simulink library "ddm"  (R2021b)
settings: Solver=VariableStepAuto  StartTime=0.0  StopTime=10.0  RelTol=1e-3
undefined symbols (not defined in the file): ADDM_FrTMTqDev_X_Nm, ADDM_RrTMTqDev_X_Nm, ENUM_ADASACCSTA_ERROR, ENUM_ADASACCSTA_OFF, ENUM_ADASACCSTA_STANDBY, ENUM_ALLOWMOV_ALLOWREADY, ENUM_APS, ENUM_BRKSTA_ERROR, ENUM_BRKSTA_OFF, ENUM_BRKSTA_ON, ENUM_BRKSW_INVALID, ENUM_BRKSW_OFF, ENUM_BRKSW_ON, ENUM_CHGPREACTERRSTA_OBCPRE, ENUM_DCDCFAULTSTA_ANYFAULTLV1, ENUM_DCDCFAULTSTA_ANYFAULTLV2, ENUM_DRIVETRAIN_AWD, ENUM_DRIVETRAIN_FWD, ENUM_DRIVETRAIN_RWD, ENUM_EDUDRTSTA_NORMAL, ENUM_EPBERROR_FAILED, ENUM_EPBSTA_APPLIED, ENUM_EPBSTA_RELEASED, ENUM_ESCAPSSta_APSUNAVAILABLE, ENUM_GEARACTUALPOSN_INVALID, ENUM_GEARACTUALPOSN_P, ENUM_HVBATTREADYPRE_READY, ENUM_HWRESETSTA_HWRESETING, ENUM_MCUWARN_LV0, ENUM_MCUWARN_LV1, ENUM_MCUWARN_LV2, ENUM_MCUWARN_LV3, ENUM_MCUWARN_NOERROR, ENUM_OBCFAULTSTA_ANYFAULT, ENUM_PAS_R2F2, ENUM_PDFAULT_BATTPDFAIL, ENUM_PDFAULT_DCDCDISABLE, ENUM_PDFAULT_MCUDISABLE, ENUM_PDFAULT_MCUDISCHRG, ENUM_POWERSTA_OFF, ENUM_POWERSTA_ON, ENUM_POWERSTA_READY, ENUM_POWERSTA_STANDBY, ENUM_PRESSINDI_LOW, ENUM_PUFAULT_BATTUPFAIL, ENUM_PUFAULT_DCDCENABLEFAIL, ENUM_PUFAULT_PRECHRGCHKFAIL, ENUM_PUFAULT_SAFETYCHKFAIL, ENUM_PWRSTASW_OFF, ENUM_PWRSTASW_OFFA, ENUM_PWRSTASW_OFFCHVCHRG, ENUM_PWRSTASW_OFFCLVCHRG, ENUM_PWRSTASW_ON, ENUM_PWRSTASW_ONHVCHRG, ENUM_PWRSTASW_READY, ENUM_PWRSTASW_STANDBY, ENUM_RAPSErrWarnSta_NORMAL, ENUM_RAPSErrWarnSta_RAPSERRLV1, ENUM_SHIFTCOMMAND_P, ENUM_SHIFTERERRSTA_PBUTTONFAILURE ... (+471)
libraries: hcu_lib x540, simulink x3
(part 7 of 26)

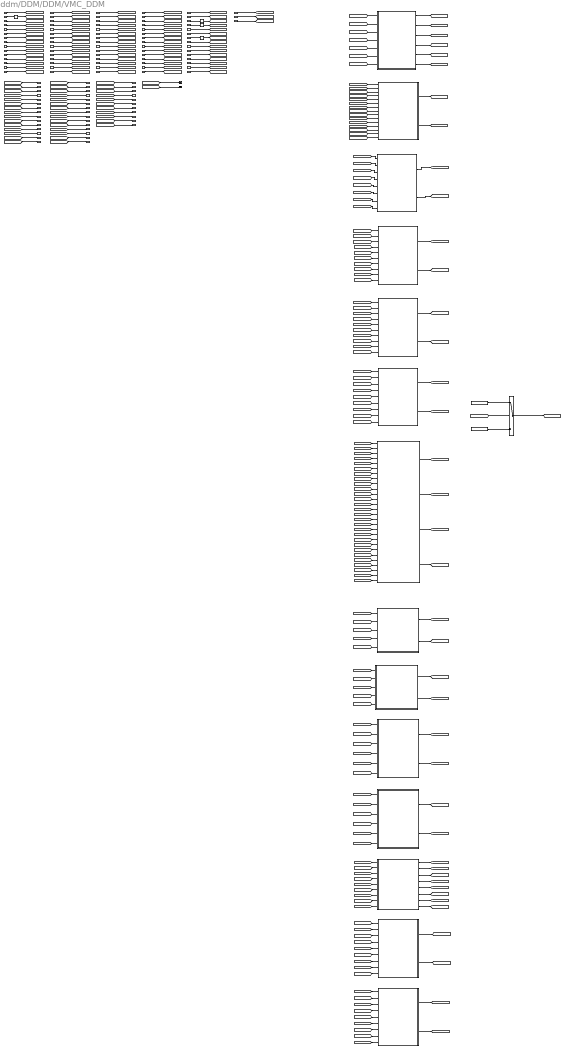
== system ddm/DDM/DDM/VMC_DDM ==
  note: No_CAN3_BUS_OFF
  note: ACC Accel
  note: CCU
  note: MCU_Rr
  note: MCU_Fr
  note: FCMACC
  note: BMS
  note: FCM1
  note: Shifter
  note: ESC
  note: Zone_dr VCU
  note: Zone_fr VCU
  note: Zone_dr
  note: Zone_fr
  note: EPS1
  task_time_s : Inport
  VDDM_FCM1NoCom_flg : Inport  Port=2
  VDDM_FCM1RCErr_flg : Inport  Port=3
  VDDM_FCM1CSErr_flg : Inport  Port=4
  VPMM_PowerSta_enum : Inport  Port=5
  VINP_ADASACCSta_enum : Inport  Port=6
  DTC_clear_request : Inport  Port=7
  VDDM_C3BMS6LCCFS_flg : Inport  Port=8
  VDDM_C3BMS6RCCFS_flg : Inport  Port=9
  VDDM_C3BMS6CSCFS_flg : Inport  Port=10
  VINP_BMSWarn8_flg : Inport  Port=11
  VINP_BMSWarn7_flg : Inport  Port=12
  VINP_BMSWarn6_flg : Inport  Port=13
  VINP_BMSWarn5_flg : Inport  Port=14
  VINP_BMSWarn4_flg : Inport  Port=15
  VINP_BMSWarn3_flg : Inport  Port=16
  VINP_VehSpeed_kph : Inport  Port=17
  VDDM_MCUF1NoComCFS_flg : Inport  Port=18
  VDDM_MCUF1RCErrCFS_flg : Inport  Port=19
  VDDM_MCUF1CSErrCFS_flg : Inport  Port=20
  VDDM_MCUWarnF_enum : Inport  Port=21
  VDDM_MCUWarnR_enum : Inport  Port=22
  VDDM_MCUR1NoComCFS_flg : Inport  Port=23
  VDDM_MCUR1RCErrCFS_flg : Inport  Port=24
  VDDM_MCUR1CSErrCFS_flg : Inport  Port=25
  VDDM_C3CCU2LCCFS_flg : Inport  Port=26
  VDDM_C3CCU2RCCFS_flg : Inport  Port=27
  VDDM_C3CCU2CSCFS_flg : Inport  Port=28
  VINP_DCDCFaultSta_enum : Inport  Port=29
  VVMC_ADASActive_flg : Inport  Port=30
  VINP_ACCRequireAccel_mps2 : Inport  Port=31
  VDDM_ESC1Err_flg : Inport  Port=32
  VDDM_ESC5Err_flg : Inport  Port=33
  VINP_ZoneSpdCtrlMode_enum : Inport  Port=34
  No_CAN1_BUS_OFF : Inport  Port=35
  No_CAN3_BUS_OFF : Inport  Port=36
  No_CAN4_BUS_OFF : Inport  Port=37
  No_CAN6_BUS_OFF : Inport  Port=38
  VTQD_ExternalTqAllow_flg : Inport  Port=39
  VTQD_ExtDoorAllow_flg : Inport  Port=40
  VINP_BMSWarn2_flg : Inport  Port=41
  VINP_BMSWarn1_flg : Inport  Port=42
  VDDM_Shifter1NoComCFS_flg : Inport  Port=43
  VDDM_Shifter1RCErrCFS_flg : Inport  Port=44
  VDDM_Shifter1CSErrCFS_flg : Inport  Port=45
  VINP_ShifterFailsta_enum : Inport  Port=46
  VTQD_GearActualPosn_enum : Inport  Port=47
  VINP_ABSFailed_flg : Inport  Port=48
  VINP_TCSFailed_flg : Inport  Port=49
  VINP_ESCFailed_flg : Inport  Port=50
  VINP_HSAFailed_flg : Inport  Port=51
  VINP_AVHFailed_flg : Inport  Port=52
  VINP_MCPressureV_flg : Inport  Port=53
  VINP_BrkSwV_flg : Inport  Port=54
  VINP_BrkPedalPosSta_flg : Inport  Port=55
  VINP_LongAccelV_flg : Inport  Port=56
  VINP_LatAccelV_flg : Inport  Port=57
  VINP_YawRateV_flg : Inport  Port=58
  VINP_LRRawWhlSpeedV_flg : Inport  Port=59
  VINP_RRRawWhlSpeedV_flg : Inport  Port=60
  VINP_LFRawWhlSpeedV_flg : Inport  Port=61
  VINP_RFRawWhlSpeedV_flg : Inport  Port=62
  VINP_CANMsgValidZoneDrVCU_flg : Inport  Port=63
  VINP_CANMsgValidZoneFrVCU_flg : Inport  Port=64
  VINP_ZoneDrMalfunLevel_enum : Inport  Port=65
  ZoneFrMalfunLevel_enum : Inport  Port=66
  VINP_CANMsgValidEPS1_flg : Inport  Port=67
  VDDM_EPSRCErr_flg : Inport  Port=68
  VDDM_EPSCSErr_flg : Inport  Port=69
  VINP_SASV_flg : Inport  Port=70
  VPMM_DrivetrainSelect_enum : Inport  Port=71
  VDDM_ClearZevDTCcmd_flg : Inport  Port=72
  VINP_FrntAxlTrqReqDrv_Nm : Inport  Port=73
  VINP_RearAxlTrqReqDrv_Nm : Inport  Port=74
  VINP_GRADE_Deg : Inport  Port=75
  VINP_FrntAxlTrqReqBrk_Nm : Inport  Port=76
  VINP_RearAxlTrqReqBrk_Nm : Inport  Port=77
  VINP_ESCAPSSta_enum : Inport  Port=78
  ACC Acceleration Command Error : Subsystem
  "BMS Signal Error " : Subsystem
  CCU Signal Error : Subsystem
  Constant4 : Constant  Value=TRUE
  Constant5 : Constant  Value=FALSE
  ESC Signal Error : Subsystem
  Enabled Subsystem : Subsystem  TreatAsAtomicUnit=on
  FCM1 : Subsystem
  FCMACC Signal Error : Subsystem
  Logical Operator : Logic  Operator=NOT  AllPortsSameDT=off  OutDataTypeStr=boolean
  Logical Operator1 : Logic  Operator=NOT  AllPortsSameDT=off  OutDataTypeStr=boolean
  MCU_Fr Signal Error : Subsystem
  MCU_Rr Signal Error : Subsystem
  NOT1 : Logic  Operator=NOT  AllPortsSameDT=off  OutDataTypeStr=boolean
  NOT21 : Logic  Operator=NOT  AllPortsSameDT=off  OutDataTypeStr=boolean
  Shifter Signal Error : Subsystem
  Switch2 : Switch  Criteria=u2 ~= 0
  Terminator1 : Terminator
  Terminator2 : Terminator
  Zone_Dr_VCU : Subsystem
  Zone_Fr_VCU : Subsystem
  Zone_dr Error : Subsystem
  Zone_fr Error : Subsystem
  VDDM_FCM1NoComDTC_raw32 : Outport
  VDDM_FCM1RCErrDTC_raw32 : Outport  Port=2
  VDDM_FCM1CSErrDTC_raw32 : Outport  Port=3
  VDDM_BMSSigErrDetDTC_raw32 : Outport  Port=4
  VDDM_FCMACCSigErrDetDTC_raw32 : Outport  Port=5
  VDDM_CCUSigErrDetDTC_raw32 : Outport  Port=6
  VDDM_ACCAccelCmdErrDetDTC_raw32 : Outport  Port=7
  VDDM_ESCSigErrDetDTC_raw32 : Outport  Port=8
  VDDM_ShifterSigErrDetDTC_raw32 : Outport  Port=9
  VDDM_DrVCUNoComDTC_raw32 : Outport  Port=10
  VDDM_FrVCUNoComDTC_raw32 : Outport  Port=11
  VDDM_ZoneDrSigErrDetDTC_raw32 : Outport  Port=12
  VDDM_ZoneFrSigErrDetDTC_raw32 : Outport  Port=13
  VDDM_EPS1NoComDTC_raw32 : Outport  Port=14
  VDDM_EPS1RCErrDTC_raw32 : Outport  Port=15
  VDDM_EPS1CSErrDTC_raw32 : Outport  Port=16
  VDDM_EPSSigErrDTC_raw32 : Outport  Port=17
  VDDM_FrMCUSigErrDetDTC_raw32 : Outport  Port=18
  VDDM_RrMCUSigErrDetDTC_raw32 : Outport  Port=19
  VDDM_FCM1NoComCFS_flg : Outport  Port=20
  VDDM_FCM1RCErrCFS_flg : Outport  Port=21
  VDDM_FCM1CSErrCFS_flg : Outport  Port=22
  VDDM_BMSSigErrCFS_flg : Outport  Port=23
  VDDM_FCMACCSigErrCFS_flg : Outport  Port=24
  VDDM_CCUSigErrCFS_flg : Outport  Port=25
  VDDM_ACCAccelCmdErrCFS_flg : Outport  Port=26
  VDDM_ESCSigErrCFS_flg : Outport  Port=27
  VDDM_ShifterSigErrCFS_flg : Outport  Port=28
  VDDM_DrVCUNoComCFS_flg : Outport  Port=29
  VDDM_FrVCUNoComCFS_flg : Outport  Port=30
  VDDM_ZoneDrSigErrCFS_flg : Outport  Port=31
  VDDM_ZoneFrSigErrCFS_flg : Outport  Port=32
  VDDM_EPS1NoComCFS_flg : Outport  Port=33
  VDDM_EPS1RCErrCFS_flg : Outport  Port=34
  VDDM_EPS1CSErrCFS_flg : Outport  Port=35
  VDDM_EPSSigErrCFS_flg : Outport  Port=36
  VDDM_FrMCUSigErrCFS_flg : Outport  Port=37
  VDDM_RrMCUSigErrCFS_flg : Outport  Port=38
  VDDM_ESC1SigErr_flg : Outport  Port=39
  VDDM_ESC5SigErr_flg : Outport  Port=40
  VDDM_EDriveSysErrVCUErrVMC_flg : Outport  Port=41
  wires:
  CCU Signal Error/2(VDDM_CCUSigErrDetDTC_raw32) -> [VDDM_CCUSigErrDetDTC_raw32]
  MCU_Rr Signal Error/2(VDDM_RrMCUSigErrDetDTC_raw32) -> [VDDM_RrMCUSigErrDetDTC_raw32]
  "BMS Signal Error "/2(VDDM_BMSSigErrDetDTC_raw32) -> [VDDM_BMSSigErrDetDTC_raw32]
  No_CAN1_BUS_OFF/1 -> [No_CAN1_BUS_OFF]
  No_CAN3_BUS_OFF/1 -> [No_CAN3_BUS_OFF]
  No_CAN4_BUS_OFF/1 -> [No_CAN4_BUS_OFF]
  VINP_ZoneSpdCtrlMode_enum/1 -> [VINP_ZoneSpdCtrlMode_enum]
  VDDM_ESC5Err_flg/1 -> [VDDM_ESC5Err_flg]
  VDDM_ESC1Err_flg/1 -> [VDDM_ESC1Err_flg]
  VINP_ACCRequireAccel_mps2/1 -> [VINP_ACCRequireAccel_mps2]
  VVMC_ADASActive_flg/1 -> [VVMC_ADASActive_flg]
  [VINP_ADASACCSta_enum] -> ACC Acceleration Command Error/9(VINP_ADASACCSta_enum)
  [VVMC_ADASActive_flg] -> ACC Acceleration Command Error/5(VVMC_ADASActive_flg)
  ACC Acceleration Command Error/1(VDDM_ACCAccelCmdErrCFS_flg) -> [VDDM_ACCAccelCmdErrCFS_flg]
  [No_CAN6_BUS_OFF] -> ACC Acceleration Command Error/6(No_CAN6_BUS_OFF)
  [VPMM_PowerSta_enum] -> ACC Acceleration Command Error/7(VPMM_PowerSta_enum)
  [DTC_clear_request] -> ACC Acceleration Command Error/10(DTC_clear_request)
  [VDDM_FCM1NoComCFS_flg] -> ACC Acceleration Command Error/2(VDDM_FCM1NoComCFS_flg)
  [VINP_ACCRequireAccel_mps2] -> ACC Acceleration Command Error/8(VINP_ACCRequireAccel_mps2)
  [VDDM_FCM1RCErrCFS_flg] -> ACC Acceleration Command Error/3(VDDM_FCM1RCErrCFS_flg)
  [VDDM_FCM1CSErrCFS_flg] -> ACC Acceleration Command Error/4(VDDM_FCM1CSErrCFS_flg)
  [task_time_s] -> ACC Acceleration Command Error/1(task_time_s)
  VINP_DCDCFaultSta_enum/1 -> [VINP_DCDCFaultSta_enum]
  VDDM_C3CCU2CSCFS_flg/1 -> [VDDM_C3CCU2CSCFS_flg]
  VDDM_C3CCU2RCCFS_flg/1 -> [VDDM_C3CCU2RCCFS_flg]
  VDDM_C3CCU2LCCFS_flg/1 -> [VDDM_C3CCU2LCCFS_flg]
  CCU Signal Error/1(VDDM_CCUSigErrCFS_flg) -> [VDDM_CCUSigErrCFS_flg]
  [VDDM_C3CCU2LCCFS_flg] -> CCU Signal Error/2(VDDM_C3CCU2LCCFS_flg)
  [task_time_s] -> CCU Signal Error/1(task_time_s)
  [VINP_DCDCFaultSta_enum] -> CCU Signal Error/7(VINP_DCDCFaultSta_enum)
  [VDDM_C3CCU2RCCFS_flg] -> CCU Signal Error/3(VDDM_C3CCU2RCCFS_flg)
  [VDDM_C3CCU2CSCFS_flg] -> CCU Signal Error/4(VDDM_C3CCU2CSCFS_flg)
  [VDDM_ClearZevDTCcmd_flg] -> CCU Signal Error/8(DTC_clear_request)
  [VPMM_PowerSta_enum] -> CCU Signal Error/6(VPMM_PowerSta_enum)
  [No_CAN3_BUS_OFF] -> CCU Signal Error/5(No_CAN3_BUS_OFF)
  VDDM_MCUR1CSErrCFS_flg/1 -> [VDDM_MCUR1CSErrCFS_flg]
  VDDM_MCUR1RCErrCFS_flg/1 -> [VDDM_MCUR1RCErrCFS_flg]
  VDDM_MCUR1NoComCFS_flg/1 -> [VDDM_MCUR1NoComCFS_flg]
  VDDM_MCUWarnR_enum/1 -> [VDDM_MCUWarnR_enum]
  [task_time_s] -> MCU_Rr Signal Error/1(task_time_s)
  [VDDM_MCUR1RCErrCFS_flg] -> MCU_Rr Signal Error/3(VDDM_MCUR1RCErrCFS_flg)
  [VDDM_MCUR1NoComCFS_flg] -> MCU_Rr Signal Error/2(VDDM_MCUR1NoComCFS_flg)
  MCU_Rr Signal Error/1(VDDM_RrMCUSigErrCFS_flg) -> [VDDM_RrMCUSigErrCFS_flg]
  [VPMM_PowerSta_enum] -> MCU_Rr Signal Error/6(VPMM_PowerSta_enum)
  [VDDM_MCUWarnR_enum] -> MCU_Rr Signal Error/7(VDDM_MCUWarnR_enum)
  [VDDM_MCUR1CSErrCFS_flg] -> MCU_Rr Signal Error/4(VDDM_MCUR1CSErrCFS_flg)
  [VDDM_ClearZevDTCcmd_flg] -> MCU_Rr Signal Error/8(DTC_clear_request)
  [No_CAN3_BUS_OFF] -> MCU_Rr Signal Error/5(No_CAN3_BUS_OFF)
  VDDM_MCUWarnF_enum/1 -> [VDDM_MCUWarnF_enum]
  VDDM_MCUF1CSErrCFS_flg/1 -> [VDDM_MCUF1CSErrCFS_flg]
  VDDM_MCUF1RCErrCFS_flg/1 -> [VDDM_MCUF1RCErrCFS_flg]
  VDDM_MCUF1NoComCFS_flg/1 -> [VDDM_MCUF1NoComCFS_flg]
  MCU_Fr Signal Error/1(VDDM_FrMCUSigErrCFS_flg) -> [VDDM_FrMCUSigErrCFS_flg]
  [VDDM_MCUF1NoComCFS_flg] -> MCU_Fr Signal Error/2(VDDM_MCUF1NoComCFS_flg)
  [VDDM_MCUWarnF_enum] -> MCU_Fr Signal Error/7(VDDM_MCUWarnF_enum)
  [VDDM_MCUF1RCErrCFS_flg] -> MCU_Fr Signal Error/3(VDDM_MCUF1RCErrCFS_flg)
  [VPMM_PowerSta_enum] -> MCU_Fr Signal Error/6(VPMM_PowerSta_enum)
  [task_time_s] -> MCU_Fr Signal Error/1(task_time_s)
  [VDDM_MCUF1CSErrCFS_flg] -> MCU_Fr Signal Error/4(VDDM_MCUF1CSErrCFS_flg)
  [No_CAN3_BUS_OFF] -> MCU_Fr Signal Error/5(No_CAN3_BUS_OFF)
  [VINP_ADASACCSta_enum] -> FCMACC Signal Error/7(VINP_ADASACCSta_enum)
  [VDDM_FCM1CSErrCFS_flg] -> FCMACC Signal Error/4(VDDM_FCM1CSErrCFS_flg)
  [VDDM_FCM1NoComCFS_flg] -> FCMACC Signal Error/2(VDDM_FCM1NoComCFS_flg)
  [DTC_clear_request] -> FCMACC Signal Error/8(DTC_clear_request)
  [task_time_s] -> FCMACC Signal Error/1(task_time_s)
  [VPMM_PowerSta_enum] -> FCMACC Signal Error/6(VPMM_PowerSta_enum)
  [No_CAN6_BUS_OFF] -> FCMACC Signal Error/5(No_CAN6_BUS_OFF)
  VINP_VehSpeed_kph/1 -> [VINP_VehSpeed_kph]
  [VDDM_ShifterSigErrCFS_flg] -> Switch2/2
  Switch2/1 -> [VDDM_EDriveSysErrVCUErrVMC_flg]
  Constant4/1 -> Switch2/1
  Constant5/1 -> Switch2/3
  [VDDM_ACCAccelCmdErrDetDTC_raw32] -> VDDM_ACCAccelCmdErrDetDTC_raw32/1
  [VDDM_FCMACCSigErrDetDTC_raw32] -> VDDM_FCMACCSigErrDetDTC_raw32/1
  [VDDM_CCUSigErrDetDTC_raw32] -> VDDM_CCUSigErrDetDTC_raw32/1
  [VDDM_BMSSigErrDetDTC_raw32] -> VDDM_BMSSigErrDetDTC_raw32/1
  [VDDM_FCM1RCErrDTC_raw32] -> VDDM_FCM1RCErrDTC_raw32/1
  [VDDM_FCM1NoComDTC_raw32] -> VDDM_FCM1NoComDTC_raw32/1
  [VDDM_FCM1CSErrDTC_raw32] -> VDDM_FCM1CSErrDTC_raw32/1
  task_time_s/1 -> [task_time_s]
  VDDM_C3BMS6RCCFS_flg/1 -> [VDDM_C3BMS6RCCFS_flg]
  VINP_BMSWarn4_flg/1 -> [VINP_BMSWarn4_flg]
  DTC_clear_request/1 -> [DTC_clear_request]
  [DTC_clear_request] -> FCM1/7(DTC_clear_request)
  [VPMM_PowerSta_enum] -> FCM1/6(VPMM_PowerSta_enum)
  [task_time_s] -> FCM1/1(task_time_s)
  [VDDM_FCM1CSErr_flg] -> FCM1/4(VDDM_FCM1CSErr_flg)
  VINP_BMSWarn8_flg/1 -> [VINP_BMSWarn8_flg]
  [VINP_BMSWarn6_flg] -> "BMS Signal Error "/9(VINP_BMSWarn6_flg)
  [VDDM_FCM1NoCom_flg] -> FCM1/2(VDDM_FCM1NoCom_flg)
  [No_CAN6_BUS_OFF] -> FCM1/5(No_CAN6_BUS_OFF)
  [VDDM_FCM1RCErr_flg] -> FCM1/3(VDDM_FCM1RCErr_flg)
  "BMS Signal Error "/1(VDDM_BMSSigErrCFS_flg) -> [VDDM_BMSSigErrCFS_flg]
  VDDM_FCM1CSErr_flg/1 -> [VDDM_FCM1CSErr_flg]
  VINP_BMSWarn6_flg/1 -> [VINP_BMSWarn6_flg]
  VINP_ADASACCSta_enum/1 -> [VINP_ADASACCSta_enum]
  VINP_BMSWarn5_flg/1 -> [VINP_BMSWarn5_flg]
  VDDM_C3BMS6LCCFS_flg/1 -> [VDDM_C3BMS6LCCFS_flg]
  [VDDM_C3BMS6LCCFS_flg] -> "BMS Signal Error "/2(VDDM_C3BMS6LCCFS_flg)
  [VDDM_C3BMS6CSCFS_flg] -> "BMS Signal Error "/4(VDDM_C3BMS6CSCFS_flg)
  [No_CAN3_BUS_OFF] -> "BMS Signal Error "/5(No_CAN3_BUS_OFF)
  [VDDM_C3BMS6RCCFS_flg] -> "BMS Signal Error "/3(VDDM_C3BMS6RCCFS_flg)
  [VINP_BMSWarn8_flg] -> "BMS Signal Error "/7(VINP_BMSWarn8_flg)
  [VINP_BMSWarn7_flg] -> "BMS Signal Error "/8(VINP_BMSWarn7_flg)
  [VPMM_PowerSta_enum] -> "BMS Signal Error "/6(VPMM_PowerSta_enum)
  [VDDM_ClearZevDTCcmd_flg] -> "BMS Signal Error "/15(DTC_clear_request)
  [VINP_BMSWarn4_flg] -> "BMS Signal Error "/11(VINP_BMSWarn4_flg)
  [VINP_BMSWarn5_flg] -> "BMS Signal Error "/10(VINP_BMSWarn5_flg)
  VDDM_FCM1NoCom_flg/1 -> Logical Operator1/1
  [task_time_s] -> "BMS Signal Error "/1(task_time_s)
  VINP_BMSWarn7_flg/1 -> [VINP_BMSWarn7_flg]
  VPMM_PowerSta_enum/1 -> [VPMM_PowerSta_enum]
  VDDM_FCM1RCErr_flg/1 -> [VDDM_FCM1RCErr_flg]
  VDDM_C3BMS6CSCFS_flg/1 -> [VDDM_C3BMS6CSCFS_flg]
  FCM1/6(VDDM_FCM1CSErrDTC_raw32) -> [VDDM_FCM1CSErrDTC_raw32]  "VDDM_FCM1CSErrDTC_raw32"
  FCM1/5(VDDM_FCM1RCErrDTC_raw32) -> [VDDM_FCM1RCErrDTC_raw32]  "VDDM_FCM1RCErrDTC_raw32"
  FCM1/4(VDDM_FCM1NoComDTC_raw32) -> [VDDM_FCM1NoComDTC_raw32]  "VDDM_FCM1NoComDTC_raw32"
  No_CAN6_BUS_OFF/1 -> [No_CAN6_BUS_OFF]
  FCM1/1(VDDM_FCM1NoComCFS_flg) -> [VDDM_FCM1NoComCFS_flg]
  FCM1/2(VDDM_FCM1RCErrCFS_flg) -> [VDDM_FCM1RCErrCFS_flg]
  FCM1/3(VDDM_FCM1CSErrCFS_flg) -> [VDDM_FCM1CSErrCFS_flg]
  [VINP_BMSWarn3_flg] -> "BMS Signal Error "/12(VINP_BMSWarn3_flg)
  [VINP_BMSWarn2_flg] -> "BMS Signal Error "/13(VINP_BMSWarn2_flg)
  [VINP_BMSWarn1_flg] -> "BMS Signal Error "/14(VINP_BMSWarn1_flg)
  [VDDM_FCM1RCErrCFS_flg] -> FCMACC Signal Error/3(VDDM_FCM1RCErrCFS_flg)
  [VTQD_ExternalTqAllow_flg] -> FCMACC Signal Error/9(VTQD_ExternalTqAllow_flg)
  [VTQD_ExtDoorAllow_flg] -> FCMACC Signal Error/10(VTQD_ExtDoorAllow_flg)
  VTQD_ExternalTqAllow_flg/1 -> [VTQD_ExternalTqAllow_flg]
  VTQD_ExtDoorAllow_flg/1 -> [VTQD_ExtDoorAllow_flg]
  VINP_BMSWarn3_flg/1 -> [VINP_BMSWarn3_flg]
  VINP_BMSWarn2_flg/1 -> [VINP_BMSWarn2_flg]
  VINP_BMSWarn1_flg/1 -> [VINP_BMSWarn1_flg]
  FCMACC Signal Error/1(VDDM_FCMACCSigErrCFS_flg) -> [VDDM_FCMACCSigErrCFS_flg]
  FCMACC Signal Error/2(VDDM_FCMACCSigErrDetDTC_raw32) -> [VDDM_FCMACCSigErrDetDTC_raw32]
  ACC Acceleration Command Error/2(VDDM_ACCAccelCmdErrDetDTC_raw32) -> [VDDM_ACCAccelCmdErrDetDTC_raw32]
  [No_CAN3_BUS_OFF] -> Shifter Signal Error/5(No_CAN3_BUS_OFF)
  [VINP_ShifterFailsta_enum] -> Shifter Signal Error/7(VINP_ShifterFailsta_enum)
  [VDDM_ClearZevDTCcmd_flg] -> Shifter Signal Error/8(DTC_clear_request)
  Shifter Signal Error/1(VDDM_ShifterSigErrCFS_flg) -> [VDDM_ShifterSigErrCFS_flg]
  Shifter Signal Error/2(VDDM_ShifterSigErrDetDTC_raw32) -> [VDDM_ShifterSigErrDetDTC_raw32]  "VDDM_ShifterSigErrDetDTC_raw32"
  [task_time_s] -> Shifter Signal Error/1(task_time_s)
  [VDDM_Shifter1RCErrCFS_flg] -> Shifter Signal Error/3(VDDM_Shifter1RCErrCFS_flg)
  [VPMM_PowerSta_enum] -> Shifter Signal Error/6(VPMM_PowerSta_enum)
  [VDDM_Shifter1NoComCFS_flg] -> Shifter Signal Error/2(VDDM_Shifter1NoComCFS_flg)
  [VDDM_Shifter1CSErrCFS_flg] -> Shifter Signal Error/4(VDDM_Shifter1CSErrCFS_flg)
  [VTQD_GearActualPosn_enum] -> Shifter Signal Error/9(VTQD_GearActualPosn_enum)
  VDDM_Shifter1NoComCFS_flg/1 -> [VDDM_Shifter1NoComCFS_flg]
  VDDM_Shifter1RCErrCFS_flg/1 -> [VDDM_Shifter1RCErrCFS_flg]
  VDDM_Shifter1CSErrCFS_flg/1 -> [VDDM_Shifter1CSErrCFS_flg]
  VINP_ShifterFailsta_enum/1 -> [VINP_ShifterFailsta_enum]
  VTQD_GearActualPosn_enum/1 -> [VTQD_GearActualPosn_enum]
  [VDDM_ClearZevDTCcmd_flg] -> ESC Signal Error/4(DTC_clear_request)
  ESC Signal Error/1(VDDM_ESCSigErrCFS_flg) -> [VDDM_ESCSigErrCFS_flg]
  [VINP_BrkSwV_flg] -> ESC Signal Error/11(VINP_BrkSwV_flg)
  [VINP_RFRawWhlSpeedV_flg] -> ESC Signal Error/19(VINP_RFRawWhlSpeedV_flg)
  [task_time_s] -> ESC Signal Error/1(task_time_s)
  [VINP_LongAccelV_flg] -> ESC Signal Error/13(VINP_LongAccelV_flg)
  ESC Signal Error/2(VDDM_ESCSigErrDetDTC_raw32) -> [VDDM_ESCSigErrDetDTC_raw32]
  [VINP_LatAccelV_flg] -> ESC Signal Error/14(VINP_LatAccelV_flg)
  [VPMM_PowerSta_enum] -> ESC Signal Error/3(VPMM_PowerSta_enum)
  [VINP_HSAFailed_flg] -> ESC Signal Error/8(VINP_HSAFailed_flg)
  [VINP_YawRateV_flg] -> ESC Signal Error/15(VINP_YawRateV_flg)
  [VINP_ABSFailed_flg] -> ESC Signal Error/5(VINP_ABSFailed_flg)
  [VINP_BrkPedalPosSta_flg] -> ESC Signal Error/12(VINP_BrkPedalPosSta_flg)
  [VINP_MCPressureV_flg] -> ESC Signal Error/10(VINP_MCPressureV_flg)
  [VINP_AVHFailed_flg] -> ESC Signal Error/9(VINP_AVHFailed_flg)
  [VINP_TCSFailed_flg] -> ESC Signal Error/6(VINP_TCSFailed_flg)
  ESC Signal Error/3(VDDM_ESC1SigErr_flg) -> [VDDM_ESC1SigErr_flg]
  [VINP_ESCFailed_flg] -> ESC Signal Error/7(VINP_ESCFailed_flg)
  [VINP_LRRawWhlSpeedV_flg] -> ESC Signal Error/16(VINP_LRRawWhlSpeedV_flg)
  [VINP_RRRawWhlSpeedV_flg] -> ESC Signal Error/17(VINP_RRRawWhlSpeedV_flg)
  [VINP_LFRawWhlSpeedV_flg] -> ESC Signal Error/18(VINP_LFRawWhlSpeedV_flg)
  ESC Signal Error/4(VDDM_ESC5SigErr_flg) -> [VDDM_ESC5SigErr_flg]
  [No_CAN1_BUS_OFF] -> ESC Signal Error/2(No_CAN1_BUS_OFF)
  VINP_ABSFailed_flg/1 -> [VINP_ABSFailed_flg]
  VINP_TCSFailed_flg/1 -> [VINP_TCSFailed_flg]
  VINP_ESCFailed_flg/1 -> [VINP_ESCFailed_flg]
  VINP_HSAFailed_flg/1 -> [VINP_HSAFailed_flg]
  VINP_AVHFailed_flg/1 -> [VINP_AVHFailed_flg]
  VINP_MCPressureV_flg/1 -> [VINP_MCPressureV_flg]
  VINP_BrkSwV_flg/1 -> [VINP_BrkSwV_flg]
  VINP_BrkPedalPosSta_flg/1 -> [VINP_BrkPedalPosSta_flg]
  VINP_LongAccelV_flg/1 -> [VINP_LongAccelV_flg]
  VINP_LatAccelV_flg/1 -> [VINP_LatAccelV_flg]
  VINP_YawRateV_flg/1 -> [VINP_YawRateV_flg]
  VINP_LRRawWhlSpeedV_flg/1 -> [VINP_LRRawWhlSpeedV_flg]
  VINP_RRRawWhlSpeedV_flg/1 -> [VINP_RRRawWhlSpeedV_flg]
  VINP_LFRawWhlSpeedV_flg/1 -> [VINP_LFRawWhlSpeedV_flg]
  VINP_RFRawWhlSpeedV_flg/1 -> [VINP_RFRawWhlSpeedV_flg]
  [task_time_s] -> Zone_Dr_VCU/1(task_time_s)
  [VPMM_PowerSta_enum] -> Zone_Dr_VCU/2(VPMM_PowerSta_enum)
  [No_CAN4_BUS_OFF] -> Zone_Dr_VCU/3(No_CAN4_BUS_OFF)
  [VDDM_DrVCUNoCom_flg] -> Zone_Dr_VCU/4(VDDM_DrVCUNoCom_flg)
  VINP_CANMsgValidZoneDrVCU_flg/1 -> Logical Operator/1
  Logical Operator/1 -> [VDDM_DrVCUNoCom_flg]
  NOT21/1 -> [VDDM_FrVCUNoCom_flg]
  VINP_CANMsgValidZoneFrVCU_flg/1 -> NOT21/1
  Zone_Dr_VCU/1(VDDM_DrVCUNoComCFS_flg) -> [VDDM_DrVCUNoComCFS_flg]
  Zone_Dr_VCU/2(VDDM_DrVCUNoComDTC_raw32) -> [VDDM_DrVCUNoComDTC_raw32]
  [VDDM_ESCSigErrDetDTC_raw32] -> VDDM_ESCSigErrDetDTC_raw32/1
  [VDDM_ShifterSigErrDetDTC_raw32] -> VDDM_ShifterSigErrDetDTC_raw32/1
  [VDDM_DrVCUNoComDTC_raw32] -> VDDM_DrVCUNoComDTC_raw32/1
  [task_time_s] -> Zone_Fr_VCU/1(task_time_s)
  [VPMM_PowerSta_enum] -> Zone_Fr_VCU/2(VPMM_PowerSta_enum)
  [No_CAN4_BUS_OFF] -> Zone_Fr_VCU/3(No_CAN4_BUS_OFF)
  [VDDM_FrVCUNoCom_flg] -> Zone_Fr_VCU/4(VDDM_FrVCUNoCom_flg)
  [VDDM_ClearZevDTCcmd_flg] -> Zone_Fr_VCU/5(DTC_clear_request)
  Zone_Fr_VCU/1(VDDM_FrVCUNoComCFS_flg) -> [VDDM_FrVCUNoComCFS_flg]
  [VDDM_FrVCUNoComDTC_raw32] -> VDDM_FrVCUNoComDTC_raw32/1
  Zone_Fr_VCU/2(VDDM_FrVCUNoComDTC_raw32) -> [VDDM_FrVCUNoComDTC_raw32]
  [task_time_s] -> Zone_dr Error/1(task_time_s)
  [VDDM_DrVCUNoComCFS_flg] -> Zone_dr Error/2(VDDM_DrVCUNoComCFS_flg)
  [No_CAN4_BUS_OFF] -> Zone_dr Error/3(No_CAN4_BUS_OFF)
  [VPMM_PowerSta_enum] -> Zone_dr Error/4(VPMM_PowerSta_enum)
  [VINP_ZoneDrMalfunLevel_enum] -> Zone_dr Error/5(VINP_ZoneDrMalfunLevel_enum)
  VINP_ZoneDrMalfunLevel_enum/1 -> [VINP_ZoneDrMalfunLevel_enum]
  ZoneFrMalfunLevel_enum/1 -> [ZoneFrMalfunLevel_enum]
  [DTC_clear_request] -> Zone_dr Error/6(DTC_clear_request)
  Zone_dr Error/1(VDDM_ZoneDrSigErrCFS_flg) -> [VDDM_ZoneDrSigErrCFS_flg]
  Zone_dr Error/2(VDDM_ZoneDrSigErrDetDTC_raw32) -> [VDDM_ZoneDrSigErrDetDTC_raw32]
  [VDDM_ZoneDrSigErrDetDTC_raw32] -> VDDM_ZoneDrSigErrDetDTC_raw32/1
  [task_time_s] -> Zone_fr Error/1(task_time_s)
  [VDDM_FrVCUNoComCFS_flg] -> Zone_fr Error/2(VDDM_FrVCUNoComCFS_flg)
  [No_CAN4_BUS_OFF] -> Zone_fr Error/3(No_CAN4_BUS_OFF)
  [VPMM_PowerSta_enum] -> Zone_fr Error/4(VPMM_PowerSta_enum)
  [ZoneFrMalfunLevel_enum] -> Zone_fr Error/5(ZoneFrMalfunLevel_enum)
  [DTC_clear_request] -> Zone_fr Error/6(DTC_clear_request)
  Zone_fr Error/1(VDDM_ZoneFrSigErrCFS_flg) -> [VDDM_ZoneFrSigErrCFS_flg]
  Zone_fr Error/2(VDDM_ZoneFrSigErrDetDTC_raw32) -> [VDDM_ZoneFrSigErrDetDTC_raw32]
  [VDDM_ZoneFrSigErrDetDTC_raw32] -> VDDM_ZoneFrSigErrDetDTC_raw32/1
  Enabled Subsystem/2(VDDM_EPS1NoComDTC_raw32) -> [VDDM_EPS1NoComDTC_raw32]
  [VDDM_EPS1NoComDTC_raw32] -> VDDM_EPS1NoComDTC_raw32/1
  Enabled Subsystem/1(VDDM_EPS1NoComCFS_flg) -> [VDDM_EPS1NoComCFS_flg]
  Enabled Subsystem/3(VDDM_EPS1RCErrCFS_flg) -> [VDDM_EPS1RCErrCFS_flg]
  Enabled Subsystem/4(VDDM_EPS1RCErrDTC_raw32) -> [VDDM_EPS1RCErrDTC_raw32]
  [VDDM_EPS1RCErrDTC_raw32] -> VDDM_EPS1RCErrDTC_raw32/1
  Enabled Subsystem/5(VDDM_EPS1CSErrCFS_flg) -> [VDDM_EPS1CSErrCFS_flg]
  Enabled Subsystem/6(VDDM_EPS1CSErrDTC_raw32) -> [VDDM_EPS1CSErrDTC_raw32]
  [VDDM_EPS1CSErrDTC_raw32] -> VDDM_EPS1CSErrDTC_raw32/1
  Enabled Subsystem/7(VDDM_EPSSigErrCFS_flg) -> [VDDM_EPSSigErrCFS_flg]
  Enabled Subsystem/8(VDDM_EPSSigErrDTC_raw32) -> [VDDM_EPSSigErrDTC_raw32]
  [VDDM_EPSSigErrDTC_raw32] -> VDDM_EPSSigErrDTC_raw32/1
  [task_time_s] -> Enabled Subsystem/1(task_time_s)
  [VPMM_PowerSta_enum] -> Enabled Subsystem/2(VPMM_PowerSta_enum)
  [VDDM_EPS1NoCom_flg] -> Enabled Subsystem/3(VDDM_EPS1NoCom_flg)
  VINP_CANMsgValidEPS1_flg/1 -> NOT1/1
  NOT1/1 -> [VDDM_EPS1NoCom_flg]
  [No_CAN1_BUS_OFF] -> Enabled Subsystem/4(No_CAN1_BUS_OFF)
  [DTC_clear_request] -> Enabled Subsystem/5(DTC_clear_request)
  [VTQD_GearActualPosn_enum] -> Enabled Subsystem/6(VTQD_GearActualPosn_enum)
  [VDDM_EPSRCErr_flg] -> Enabled Subsystem/7(VDDM_EPSRCErr_flg)
  VDDM_EPSRCErr_flg/1 -> [VDDM_EPSRCErr_flg]
  [VDDM_EPSCSErr_flg] -> Enabled Subsystem/8(VDDM_EPSCSErr_flg)
  VDDM_EPSCSErr_flg/1 -> [VDDM_EPSCSErr_flg]
  [VINP_SASV_flg] -> Enabled Subsystem/9(VINP_SASV_flg)
  VINP_SASV_flg/1 -> [VINP_SASV_flg]
  MCU_Fr Signal Error/2(VDDM_FrMCUSigErrDetDTC_raw32) -> [VDDM_FrMCUSigErrDetDTC_raw32]
  [VDDM_ClearZevDTCcmd_flg] -> MCU_Fr Signal Error/8(DTC_clear_request)
  [VPMM_DrivetrainSelect_enum] -> MCU_Fr Signal Error/9(VPMM_DrivetrainSelect_enum)
  VPMM_DrivetrainSelect_enum/1 -> [VPMM_DrivetrainSelect_enum]
  [VPMM_DrivetrainSelect_enum] -> MCU_Rr Signal Error/9(VPMM_DrivetrainSelect_enum)
  [VDDM_FrMCUSigErrDetDTC_raw32] -> VDDM_FrMCUSigErrDetDTC_raw32/1
  [VDDM_RrMCUSigErrDetDTC_raw32] -> VDDM_RrMCUSigErrDetDTC_raw32/1
  [VDDM_FCM1NoComCFS_flg] -> VDDM_FCM1NoComCFS_flg/1
  [VDDM_FCM1RCErrCFS_flg] -> VDDM_FCM1RCErrCFS_flg/1
  [VDDM_FCM1CSErrCFS_flg] -> VDDM_FCM1CSErrCFS_flg/1
  [VDDM_BMSSigErrCFS_flg] -> VDDM_BMSSigErrCFS_flg/1
  [VDDM_FCMACCSigErrCFS_flg] -> VDDM_FCMACCSigErrCFS_flg/1
  [VDDM_CCUSigErrCFS_flg] -> VDDM_CCUSigErrCFS_flg/1
  [VDDM_ACCAccelCmdErrCFS_flg] -> VDDM_ACCAccelCmdErrCFS_flg/1
  [VDDM_ESCSigErrCFS_flg] -> VDDM_ESCSigErrCFS_flg/1
  [VDDM_ShifterSigErrCFS_flg] -> VDDM_ShifterSigErrCFS_flg/1
  [VDDM_DrVCUNoComCFS_flg] -> VDDM_DrVCUNoComCFS_flg/1
  [VDDM_FrVCUNoComCFS_flg] -> VDDM_FrVCUNoComCFS_flg/1
  [VDDM_ZoneDrSigErrCFS_flg] -> VDDM_ZoneDrSigErrCFS_flg/1
  [VDDM_ZoneFrSigErrCFS_flg] -> VDDM_ZoneFrSigErrCFS_flg/1
  [VDDM_EPS1NoComCFS_flg] -> VDDM_EPS1NoComCFS_flg/1
  [VDDM_EPS1RCErrCFS_flg] -> VDDM_EPS1RCErrCFS_flg/1
  [VDDM_EPS1CSErrCFS_flg] -> VDDM_EPS1CSErrCFS_flg/1
  [VDDM_EPSSigErrCFS_flg] -> VDDM_EPSSigErrCFS_flg/1
  [VDDM_FrMCUSigErrCFS_flg] -> VDDM_FrMCUSigErrCFS_flg/1
  [VDDM_RrMCUSigErrCFS_flg] -> VDDM_RrMCUSigErrCFS_flg/1
  [VDDM_ESC5SigErr_flg] -> VDDM_ESC5SigErr_flg/1
  [VDDM_ESC1SigErr_flg] -> VDDM_ESC1SigErr_flg/1
  Logical Operator1/1 -> [VDDM_FCM1NoCom_flg]
  [VDDM_EDriveSysErrVCUErrVMC_flg] -> VDDM_EDriveSysErrVCUErrVMC_flg/1
  [VINP_ZoneSpdCtrlMode_enum] -> Terminator1/1
  [VINP_VehSpeed_kph] -> Terminator2/1
  VDDM_ClearZevDTCcmd_flg/1 -> [VDDM_ClearZevDTCcmd_flg]
  [VDDM_ClearZevDTCcmd_flg] -> Zone_Dr_VCU/5(DTC_clear_request)
  [VINP_VehSpeed_kph] -> ESC Signal Error/20(VINP_VehSpeed_kph)
  [VINP_FrntAxlTrqReqDrv_Nm] -> ESC Signal Error/21(VINP_FrntAxlTrqReqDrv_Nm)
  [VINP_RearAxlTrqReqDrv_Nm] -> ESC Signal Error/22(VINP_RearAxlTrqReqDrv_Nm)
  [VDDM_ESC1Err_flg] -> ESC Signal Error/23(VDDM_ESC1Err_flg)
  [VDDM_ESC5Err_flg] -> ESC Signal Error/24(VDDM_ESC5Err_flg)
  [VINP_GRADE_Deg] -> ESC Signal Error/25(VINP_GRADE_Deg)
  [VINP_FrntAxlTrqReqBrk_Nm] -> ESC Signal Error/26(VINP_FrntAxlTrqReqBrk_Nm)
  [VINP_RearAxlTrqReqBrk_Nm] -> ESC Signal Error/27(VINP_RearAxlTrqReqBrk_Nm)
  [VINP_ESCAPSSta_enum] -> ESC Signal Error/28(VINP_ESCAPSSta_enum)
  VINP_FrntAxlTrqReqDrv_Nm/1 -> [VINP_FrntAxlTrqReqDrv_Nm]
  VINP_GRADE_Deg/1 -> [VINP_GRADE_Deg]
  VINP_RearAxlTrqReqDrv_Nm/1 -> [VINP_RearAxlTrqReqDrv_Nm]
  VINP_ESCAPSSta_enum/1 -> [VINP_ESCAPSSta_enum]
  VINP_RearAxlTrqReqBrk_Nm/1 -> [VINP_RearAxlTrqReqBrk_Nm]
  VINP_FrntAxlTrqReqBrk_Nm/1 -> [VINP_FrntAxlTrqReqBrk_Nm]

== system ddm/DDM/DDM_MCU_Signal_Selector/DDM Signal Convert  ==
  VINP_CANMsgValidMCUBF1_flg : Inport
  VINP_CANMsgValidMCUNF1_flg : Inport  Port=2
  VINP_MCUBF1RCErr_flg : Inport  Port=3
  VINP_MCUNF1RCErr_flg : Inport  Port=4
  VINP_MCUBF1CSErr_flg : Inport  Port=5
  VINP_MCUNF1CSErr_flg : Inport  Port=6
  VINP_CANMsgValidMCUBR1_flg : Inport  Port=7
  VINP_CANMsgValidMCUNR1_flg : Inport  Port=8
  VINP_MCUBR1RCErr_flg : Inport  Port=9
  VINP_MCUNR1RCErr_flg : Inport  Port=10
  VINP_MCUBR1CSErr_flg : Inport  Port=11
  VINP_MCUNR1CSErr_flg : Inport  Port=12
  VINP_VehicleType_enum : Inport  Port=13
  VINP_MCUWarnFNidec_enum : Inport  Port=14
  VINP_MCUWarnRNidec_enum : Inport  Port=15
  VINP_MCUWarnF_enum : Inport  Port=16
  VINP_MCUWarnR_enum : Inport  Port=17
  VINP_FrMCUReady4Pre_flg : Inport  Port=18
  VINP_FrMCUReady4PreNidec_flg : Inport  Port=19
  VINP_RrMCUReady4Pre_flg : Inport  Port=20
  VINP_RrMCUReady4PreNidec_flg : Inport  Port=21
  VINP_FrMCUEnaSta_flg : Inport  Port=22
  VINP_FrMCUEnaStaNidec_flg : Inport  Port=23
  VINP_RrMCUEnaSta_flg : Inport  Port=24
  VINP_RrMCUEnaStaNidec_flg : Inport  Port=25
  VINP_FrMCUDCBusVolt_V : Inport  Port=26
  VINP_FrMCUDCBusVoltNidec_V : Inport  Port=27
  VINP_RrMCUDCBusVolt_V : Inport  Port=28
  VINP_RrMCUDCBusVoltNidec_V : Inport  Port=29
  Constant{1..14} (14 alike) : Constant  Value=ENUM_VEHICLETYPE_D31L24
  Relational Operator{1..14} (14 alike) : RelationalOperator  Operator=~=  OutDataTypeStr=boolean  RndMeth=Simplest
  Switch{1..14} (14 alike) : Switch  Criteria=u2 ~= 0
  VDDM_CANMsgValidMCUF1_flg : Outport
  VDDM_MCUF1RCErr_flg : Outport  Port=2
  VDDM_MCUF1CSErr_flg : Outport  Port=3
  VDDM_CANMsgValidMCUR1_flg : Outport  Port=4
  VDDM_MCUR1RCErr_flg : Outport  Port=5
  VDDM_MCUR1CSErr_flg : Outport  Port=6
  VDDM_MCUWarnF_enum : Outport  Port=7
  VDDM_MCUWarnR_enum : Outport  Port=8
  VDDM_FrMCUReady4Pre_flg : Outport  Port=9
  VDDM_RrMCUReady4Pre_flg : Outport  Port=10
  VDDM_FrMCUEnaSta_flg : Outport  Port=11
  VDDM_RrMCUEnaSta_flg : Outport  Port=12
  VDDM_FrMCUDCBusVolt_V : Outport  Port=13
  VDDM_RrMCUDCBusVolt_V : Outport  Port=14
  wires:
  [VDDM_FrMCUDCBusVolt_V] -> VDDM_FrMCUDCBusVolt_V/1
  [VDDM_RrMCUDCBusVolt_V] -> VDDM_RrMCUDCBusVolt_V/1
  [VINP_RrMCUDCBusVoltNidec_V] -> Switch14/3
  [VINP_RrMCUDCBusVolt_V] -> Switch14/1
  Constant14/1 -> Relational Operator14/2
  Switch14/1 -> [VDDM_RrMCUDCBusVolt_V]  "VDDM_RrMCUDCBusVolt_V"
  [VINP_VehicleType_enum] -> Relational Operator14/1
  Relational Operator14/1 -> Switch14/2
  Relational Operator13/1 -> Switch13/2
  [VINP_VehicleType_enum] -> Relational Operator13/1
  Switch13/1 -> [VDDM_FrMCUDCBusVolt_V]  "VDDM_FrMCUDCBusVolt_V"
  Constant13/1 -> Relational Operator13/2
  [VINP_FrMCUDCBusVolt_V] -> Switch13/1
  [VINP_FrMCUDCBusVoltNidec_V] -> Switch13/3
  VINP_RrMCUDCBusVoltNidec_V/1 -> [VINP_RrMCUDCBusVoltNidec_V]
  VINP_RrMCUDCBusVolt_V/1 -> [VINP_RrMCUDCBusVolt_V]
  VINP_FrMCUDCBusVoltNidec_V/1 -> [VINP_FrMCUDCBusVoltNidec_V]
  VINP_FrMCUDCBusVolt_V/1 -> [VINP_FrMCUDCBusVolt_V]
  [VDDM_RrMCUEnaSta_flg] -> VDDM_RrMCUEnaSta_flg/1
  [VDDM_FrMCUEnaSta_flg] -> VDDM_FrMCUEnaSta_flg/1
  Relational Operator12/1 -> Switch12/2
  [VINP_VehicleType_enum] -> Relational Operator12/1
  Switch12/1 -> [VDDM_RrMCUEnaSta_flg]  "VDDM_RrMCUEnaSta_flg"
  Constant12/1 -> Relational Operator12/2
  [VINP_RrMCUEnaSta_flg] -> Switch12/1
  [VINP_RrMCUEnaStaNidec_flg] -> Switch12/3
  [VINP_FrMCUEnaStaNidec_flg] -> Switch11/3
  [VINP_FrMCUEnaSta_flg] -> Switch11/1
  Constant11/1 -> Relational Operator11/2
  Switch11/1 -> [VDDM_FrMCUEnaSta_flg]  "VDDM_FrMCUEnaSta_flg"
  [VINP_VehicleType_enum] -> Relational Operator11/1
  Relational Operator11/1 -> Switch11/2
  VINP_RrMCUEnaStaNidec_flg/1 -> [VINP_RrMCUEnaStaNidec_flg]
  VINP_RrMCUEnaSta_flg/1 -> [VINP_RrMCUEnaSta_flg]
  VINP_FrMCUEnaStaNidec_flg/1 -> [VINP_FrMCUEnaStaNidec_flg]
  VINP_FrMCUEnaSta_flg/1 -> [VINP_FrMCUEnaSta_flg]
  [VDDM_FrMCUReady4Pre_flg] -> VDDM_FrMCUReady4Pre_flg/1
  [VDDM_RrMCUReady4Pre_flg] -> VDDM_RrMCUReady4Pre_flg/1
  [VINP_RrMCUReady4PreNidec_flg] -> Switch10/3
  [VINP_RrMCUReady4Pre_flg] -> Switch10/1
  Constant4/1 -> Relational Operator10/2
  Switch10/1 -> [VDDM_RrMCUReady4Pre_flg]  "VDDM_RrMCUReady4Pre_flg"
  [VINP_VehicleType_enum] -> Relational Operator10/1
  Relational Operator10/1 -> Switch10/2
  Relational Operator9/1 -> Switch5/2
  [VINP_VehicleType_enum] -> Relational Operator9/1
  Switch5/1 -> [VDDM_FrMCUReady4Pre_flg]  "VDDM_FrMCUReady4Pre_flg"
  Constant3/1 -> Relational Operator9/2
  [VINP_FrMCUReady4Pre_flg] -> Switch5/1
  [VINP_FrMCUReady4PreNidec_flg] -> Switch5/3
  VINP_RrMCUReady4PreNidec_flg/1 -> [VINP_RrMCUReady4PreNidec_flg]
  VINP_FrMCUReady4PreNidec_flg/1 -> [VINP_FrMCUReady4PreNidec_flg]
  VINP_RrMCUReady4Pre_flg/1 -> [VINP_RrMCUReady4Pre_flg]
  VINP_FrMCUReady4Pre_flg/1 -> [VINP_FrMCUReady4Pre_flg]
  [VDDM_MCUWarnR_enum] -> VDDM_MCUWarnR_enum/1
  [VDDM_MCUWarnF_enum] -> VDDM_MCUWarnF_enum/1
  Relational Operator3/1 -> Switch4/2
  [VINP_VehicleType_enum] -> Relational Operator3/1
  Switch4/1 -> [VDDM_MCUWarnR_enum]  "VDDM_MCUWarnR_enum"
  Constant2/1 -> Relational Operator3/2
  [VINP_MCUWarnR_enum] -> Switch4/1
  [VINP_MCUWarnRNidec_enum] -> Switch4/3
  [VINP_MCUWarnFNidec_enum] -> Switch1/3
  [VINP_MCUWarnF_enum] -> Switch1/1
  Constant1/1 -> Relational Operator2/2
  Switch1/1 -> [VDDM_MCUWarnF_enum]  "VDDM_MCUWarnF_enum"
  [VINP_VehicleType_enum] -> Relational Operator2/1
  Relational Operator2/1 -> Switch1/2
  VINP_MCUWarnFNidec_enum/1 -> [VINP_MCUWarnFNidec_enum]
  VINP_MCUWarnF_enum/1 -> [VINP_MCUWarnF_enum]
  VINP_MCUWarnRNidec_enum/1 -> [VINP_MCUWarnRNidec_enum]
  VINP_MCUWarnR_enum/1 -> [VINP_MCUWarnR_enum]
  [VDDM_MCUR1CSErr_flg] -> VDDM_MCUR1CSErr_flg/1
  [VDDM_MCUR1RCErr_flg] -> VDDM_MCUR1RCErr_flg/1
  [VDDM_CANMsgValidMCUR1_flg] -> VDDM_CANMsgValidMCUR1_flg/1
  [VDDM_MCUF1CSErr_flg] -> VDDM_MCUF1CSErr_flg/1
  [VDDM_MCUF1RCErr_flg] -> VDDM_MCUF1RCErr_flg/1
  [VDDM_CANMsgValidMCUF1_flg] -> VDDM_CANMsgValidMCUF1_flg/1
  VINP_VehicleType_enum/1 -> [VINP_VehicleType_enum]
  VINP_MCUBR1CSErr_flg/1 -> [VINP_MCUBR1CSErr_flg]
  VINP_MCUNR1CSErr_flg/1 -> [VINP_MCUNR1CSErr_flg]
  VINP_MCUNR1RCErr_flg/1 -> [VINP_MCUNR1RCErr_flg]
  VINP_MCUBR1RCErr_flg/1 -> [VINP_MCUBR1RCErr_flg]
  VINP_CANMsgValidMCUNR1_flg/1 -> [VINP_CANMsgValidMCUNR1_flg]
  VINP_CANMsgValidMCUBR1_flg/1 -> [VINP_CANMsgValidMCUBR1_flg]
  VINP_MCUNF1CSErr_flg/1 -> [VINP_MCUNF1CSErr_flg]
  VINP_MCUBF1CSErr_flg/1 -> [VINP_MCUBF1CSErr_flg]
  VINP_MCUNF1RCErr_flg/1 -> [VINP_MCUNF1RCErr_flg]
  VINP_MCUBF1RCErr_flg/1 -> [VINP_MCUBF1RCErr_flg]
  VINP_CANMsgValidMCUNF1_flg/1 -> [VINP_CANMsgValidMCUNF1_flg]
  VINP_CANMsgValidMCUBF1_flg/1 -> [VINP_CANMsgValidMCUBF1_flg]
  Switch3/1 -> [VDDM_MCUF1RCErr_flg]  "VDDM_MCUF1RCErr_flg"
  Switch2/1 -> [VDDM_CANMsgValidMCUF1_flg]  "VDDM_CANMsgValidMCUF1_flg"
  Constant6/1 -> Relational Operator4/2
  Switch8/1 -> [VDDM_MCUR1RCErr_flg]  "VDDM_MCUR1RCErr_flg"
  Switch9/1 -> [VDDM_MCUR1CSErr_flg]  "VDDM_MCUR1CSErr_flg"
  Switch6/1 -> [VDDM_MCUF1CSErr_flg]  "VDDM_MCUF1CSErr_flg"
  [VINP_MCUBF1CSErr_flg] -> Switch6/1
  [VINP_VehicleType_enum] -> Relational Operator7/1
  [VINP_MCUBR1RCErr_flg] -> Switch8/1
  [VINP_MCUBR1CSErr_flg] -> Switch9/1
  [VINP_MCUNR1CSErr_flg] -> Switch9/3
  Switch7/1 -> [VDDM_CANMsgValidMCUR1_flg]  "VDDM_CANMsgValidMCUR1_flg"
  [VINP_CANMsgValidMCUNR1_flg] -> Switch7/3
  [VINP_CANMsgValidMCUBR1_flg] -> Switch7/1
  Relational Operator5/1 -> Switch6/2
  [VINP_MCUBF1RCErr_flg] -> Switch3/1
  [VINP_MCUNR1RCErr_flg] -> Switch8/3
  [VINP_MCUNF1RCErr_flg] -> Switch3/3
  [VINP_CANMsgValidMCUBF1_flg] -> Switch2/1
  [VINP_MCUNF1CSErr_flg] -> Switch6/3
  [VINP_CANMsgValidMCUNF1_flg] -> Switch2/3
  Relational Operator8/1 -> Switch9/2
  [VINP_VehicleType_enum] -> Relational Operator1/1
  Constant8/1 -> Relational Operator6/2
  [VINP_VehicleType_enum] -> Relational Operator6/1
  Constant10/1 -> Relational Operator8/2
  [VINP_VehicleType_enum] -> Relational Operator8/1
  Constant5/1 -> Relational Operator1/2
  Constant9/1 -> Relational Operator7/2
  Constant7/1 -> Relational Operator5/2
  [VINP_VehicleType_enum] -> Relational Operator5/1
  [VINP_VehicleType_enum] -> Relational Operator4/1
  Relational Operator4/1 -> Switch3/2
  Relational Operator6/1 -> Switch7/2
  Relational Operator1/1 -> Switch2/2
  Relational Operator7/1 -> Switch8/2

== system ddm/DDM/DDM/APM/Subsystem ==
  USSSta_flg : Inport
  VPMM_SysPwrSta_enum : Inport  Port=2
  VAPM_SNSRLayout_enum : Inport  Port=3
  Constant1 : Constant  Value=ENUM_PWRSTASW_READY
  Constant17 : Constant  Value=ENUM_PWRSTASW_READY
  Constant2 : Constant  Value=ENUM_PWRSTASW_ON
  Constant25 : Constant  Value=FALSE
  Constant3 : Constant  Value=ENUM_PWRSTASW_ON
  Constant4 : Constant  Value=ENUM_APS
  Constant5 : Constant  Value=ENUM_PAS_R2F2
  Equal{1..6} (6 alike) : RelationalOperator  Operator===  OutDataTypeStr=boolean  RndMeth=Simplest
  Logical Operator1 : Logic  Operator=NOT  AllPortsSameDT=off  OutDataTypeStr=boolean
  Logical Operator13 : Logic  Operator=OR  AllPortsSameDT=off  OutDataTypeStr=boolean
  Logical Operator2 : Logic  AllPortsSameDT=off  OutDataTypeStr=boolean
  Logical Operator3 : Logic  Operator=OR  AllPortsSameDT=off  OutDataTypeStr=boolean
  Logical Operator4 : Logic  AllPortsSameDT=off  OutDataTypeStr=boolean
  Logical Operator5 : Logic  Operator=OR  AllPortsSameDT=off  OutDataTypeStr=boolean
  Switch2 : Switch  Criteria=u2 ~= 0
  Pass_flg : Outport
  CFS_flg : Outport  Port=2
  wires:
  Constant5/1 -> Equal5/2
  Equal5/1 -> Logical Operator5/2
  Logical Operator5/1 -> Switch2/2
  VAPM_SNSRLayout_enum/1 -> Equal5/1, Equal4/2
  Constant4/1 -> Equal4/1
  Constant25/1 -> Switch2/3
  Equal4/1 -> Logical Operator5/1
  USSSta_flg/1 -> Switch2/1
  [VPMM_SysPwrSta_enum] -> Equal2/1
  Equal6/1 -> Logical Operator13/1
  Constant17/1 -> Equal2/2
  Constant3/1 -> Equal6/2
  Equal2/1 -> Logical Operator13/2
  [VPMM_SysPwrSta_enum] -> Equal6/1
  Logical Operator13/1 -> Logical Operator2/1
  Logical Operator1/1 -> Logical Operator2/2
  Logical Operator2/1 -> Pass_flg/1
  Logical Operator3/1 -> Logical Operator4/2
  [VPMM_SysPwrSta_enum] -> Equal3/1
  Equal1/1 -> Logical Operator3/2
  Constant2/1 -> Equal3/2
  Constant1/1 -> Equal1/2
  Equal3/1 -> Logical Operator3/1
  [VPMM_SysPwrSta_enum] -> Equal1/1
  Switch2/1 -> Logical Operator1/1, Logical Operator4/1
  Logical Operator4/1 -> CFS_flg/1
  VPMM_SysPwrSta_enum/1 -> [VPMM_SysPwrSta_enum]

== system ddm/DDM/DDM/APM/Subsystem1 ==
  USSSta_flg : Inport
  VPMM_SysPwrSta_enum : Inport  Port=2
  VAPM_SNSRLayout_enum : Inport  Port=3
  Constant1 : Constant  Value=ENUM_PWRSTASW_READY
  Constant17 : Constant  Value=ENUM_PWRSTASW_READY
  Constant2 : Constant  Value=ENUM_PWRSTASW_ON
  Constant25 : Constant  Value=FALSE
  Constant3 : Constant  Value=ENUM_PWRSTASW_ON
  Constant5 : Constant  Value=ENUM_APS
  Equal{1..3,5..6} (5 alike) : RelationalOperator  Operator===  OutDataTypeStr=boolean  RndMeth=Simplest
  Logical Operator1 : Logic  Operator=NOT  AllPortsSameDT=off  OutDataTypeStr=boolean
  Logical Operator13 : Logic  Operator=OR  AllPortsSameDT=off  OutDataTypeStr=boolean
  Logical Operator2 : Logic  AllPortsSameDT=off  OutDataTypeStr=boolean
  Logical Operator3 : Logic  Operator=OR  AllPortsSameDT=off  OutDataTypeStr=boolean
  Logical Operator4 : Logic  AllPortsSameDT=off  OutDataTypeStr=boolean
  Switch2 : Switch  Criteria=u2 ~= 0
  Pass_flg : Outport
  CFS_flg : Outport  Port=2
  wires:
  USSSta_flg/1 -> Switch2/1
  Constant25/1 -> Switch2/3
  Equal5/1 -> Switch2/2
  VAPM_SNSRLayout_enum/1 -> Equal5/1
  Constant5/1 -> Equal5/2
  VPMM_SysPwrSta_enum/1 -> [VPMM_SysPwrSta_enum]
  Logical Operator4/1 -> CFS_flg/1
  Switch2/1 -> Logical Operator1/1, Logical Operator4/1
  [VPMM_SysPwrSta_enum] -> Equal1/1
  Equal3/1 -> Logical Operator3/1
  Constant1/1 -> Equal1/2
  Constant2/1 -> Equal3/2
  Equal1/1 -> Logical Operator3/2
  [VPMM_SysPwrSta_enum] -> Equal3/1
  Logical Operator3/1 -> Logical Operator4/2
  Logical Operator2/1 -> Pass_flg/1
  Logical Operator1/1 -> Logical Operator2/2
  Logical Operator13/1 -> Logical Operator2/1
  [VPMM_SysPwrSta_enum] -> Equal6/1
  Equal2/1 -> Logical Operator13/2
  Constant3/1 -> Equal6/2
  Constant17/1 -> Equal2/2
  Equal6/1 -> Logical Operator13/1
  [VPMM_SysPwrSta_enum] -> Equal2/1

== system ddm/DDM/DDM/APM/Subsystem10 ==
  USSSta_flg : Inport
  VPMM_SysPwrSta_enum : Inport  Port=2
  VAPM_SNSRLayout_enum : Inport  Port=3
  Constant1 : Constant  Value=ENUM_PWRSTASW_READY
  Constant17 : Constant  Value=ENUM_PWRSTASW_READY
  Constant2 : Constant  Value=ENUM_PWRSTASW_ON
  Constant25 : Constant  Value=FALSE
  Constant3 : Constant  Value=ENUM_PWRSTASW_ON
  Constant5 : Constant  Value=ENUM_APS
  Equal{1..3,5..6} (5 alike) : RelationalOperator  Operator===  OutDataTypeStr=boolean  RndMeth=Simplest
  Logical Operator1 : Logic  Operator=NOT  AllPortsSameDT=off  OutDataTypeStr=boolean
  Logical Operator13 : Logic  Operator=OR  AllPortsSameDT=off  OutDataTypeStr=boolean
  Logical Operator2 : Logic  AllPortsSameDT=off  OutDataTypeStr=boolean
  Logical Operator3 : Logic  Operator=OR  AllPortsSameDT=off  OutDataTypeStr=boolean
  Logical Operator4 : Logic  AllPortsSameDT=off  OutDataTypeStr=boolean
  Switch2 : Switch  Criteria=u2 ~= 0
  Pass_flg : Outport
  CFS_flg : Outport  Port=2
  wires:
  [VPMM_SysPwrSta_enum] -> Equal2/1
  Equal6/1 -> Logical Operator13/1
  Constant17/1 -> Equal2/2
  Constant3/1 -> Equal6/2
  Equal2/1 -> Logical Operator13/2
  [VPMM_SysPwrSta_enum] -> Equal6/1
  Logical Operator13/1 -> Logical Operator2/1
  Logical Operator1/1 -> Logical Operator2/2
  Logical Operator2/1 -> Pass_flg/1
  Logical Operator3/1 -> Logical Operator4/2
  [VPMM_SysPwrSta_enum] -> Equal3/1
  Equal1/1 -> Logical Operator3/2
  Constant2/1 -> Equal3/2
  Constant1/1 -> Equal1/2
  Equal3/1 -> Logical Operator3/1
  [VPMM_SysPwrSta_enum] -> Equal1/1
  Switch2/1 -> Logical Operator4/1, Logical Operator1/1
  Logical Operator4/1 -> CFS_flg/1
  VPMM_SysPwrSta_enum/1 -> [VPMM_SysPwrSta_enum]
  Constant5/1 -> Equal5/2
  VAPM_SNSRLayout_enum/1 -> Equal5/1
  Equal5/1 -> Switch2/2
  Constant25/1 -> Switch2/3
  USSSta_flg/1 -> Switch2/1

== system ddm/DDM/DDM/APM/Subsystem11 ==
  USSSta_flg : Inport
  VPMM_SysPwrSta_enum : Inport  Port=2
  VAPM_SNSRLayout_enum : Inport  Port=3
  Constant1 : Constant  Value=ENUM_PWRSTASW_READY
  Constant17 : Constant  Value=ENUM_PWRSTASW_READY
  Constant2 : Constant  Value=ENUM_PWRSTASW_ON
  Constant25 : Constant  Value=FALSE
  Constant3 : Constant  Value=ENUM_PWRSTASW_ON
  Constant5 : Constant  Value=ENUM_APS
  Equal{1..3,5..6} (5 alike) : RelationalOperator  Operator===  OutDataTypeStr=boolean  RndMeth=Simplest
  Logical Operator1 : Logic  Operator=NOT  AllPortsSameDT=off  OutDataTypeStr=boolean
  Logical Operator13 : Logic  Operator=OR  AllPortsSameDT=off  OutDataTypeStr=boolean
  Logical Operator2 : Logic  AllPortsSameDT=off  OutDataTypeStr=boolean
  Logical Operator3 : Logic  Operator=OR  AllPortsSameDT=off  OutDataTypeStr=boolean
  Logical Operator4 : Logic  AllPortsSameDT=off  OutDataTypeStr=boolean
  Switch2 : Switch  Criteria=u2 ~= 0
  Pass_flg : Outport
  CFS_flg : Outport  Port=2
  wires:
  [VPMM_SysPwrSta_enum] -> Equal2/1
  Equal6/1 -> Logical Operator13/1
  Constant17/1 -> Equal2/2
  Constant3/1 -> Equal6/2
  Equal2/1 -> Logical Operator13/2
  [VPMM_SysPwrSta_enum] -> Equal6/1
  Logical Operator13/1 -> Logical Operator2/1
  Logical Operator1/1 -> Logical Operator2/2
  Logical Operator2/1 -> Pass_flg/1
  Logical Operator3/1 -> Logical Operator4/2
  [VPMM_SysPwrSta_enum] -> Equal3/1
  Equal1/1 -> Logical Operator3/2
  Constant2/1 -> Equal3/2
  Constant1/1 -> Equal1/2
  Equal3/1 -> Logical Operator3/1
  [VPMM_SysPwrSta_enum] -> Equal1/1
  Switch2/1 -> Logical Operator4/1, Logical Operator1/1
  Logical Operator4/1 -> CFS_flg/1
  VPMM_SysPwrSta_enum/1 -> [VPMM_SysPwrSta_enum]
  Constant5/1 -> Equal5/2
  VAPM_SNSRLayout_enum/1 -> Equal5/1
  Equal5/1 -> Switch2/2
  Constant25/1 -> Switch2/3
  USSSta_flg/1 -> Switch2/1

== system ddm/DDM/DDM/APM/Subsystem2 ==
  USSSta_flg : Inport
  VPMM_SysPwrSta_enum : Inport  Port=2
  VAPM_SNSRLayout_enum : Inport  Port=3
  Constant1 : Constant  Value=ENUM_PWRSTASW_READY
  Constant17 : Constant  Value=ENUM_PWRSTASW_READY
  Constant2 : Constant  Value=ENUM_PWRSTASW_ON
  Constant25 : Constant  Value=FALSE
  Constant3 : Constant  Value=ENUM_PWRSTASW_ON
  Constant5 : Constant  Value=ENUM_APS
  Equal{1..3,5..6} (5 alike) : RelationalOperator  Operator===  OutDataTypeStr=boolean  RndMeth=Simplest
  Logical Operator1 : Logic  Operator=NOT  AllPortsSameDT=off  OutDataTypeStr=boolean
  Logical Operator13 : Logic  Operator=OR  AllPortsSameDT=off  OutDataTypeStr=boolean
  Logical Operator2 : Logic  AllPortsSameDT=off  OutDataTypeStr=boolean
  Logical Operator3 : Logic  Operator=OR  AllPortsSameDT=off  OutDataTypeStr=boolean
  Logical Operator4 : Logic  AllPortsSameDT=off  OutDataTypeStr=boolean
  Switch2 : Switch  Criteria=u2 ~= 0
  Pass_flg : Outport
  CFS_flg : Outport  Port=2
  wires:
  [VPMM_SysPwrSta_enum] -> Equal2/1
  Equal6/1 -> Logical Operator13/1
  Constant17/1 -> Equal2/2
  Constant3/1 -> Equal6/2
  Equal2/1 -> Logical Operator13/2
  [VPMM_SysPwrSta_enum] -> Equal6/1
  Logical Operator13/1 -> Logical Operator2/1
  Logical Operator1/1 -> Logical Operator2/2
  Logical Operator2/1 -> Pass_flg/1
  Logical Operator3/1 -> Logical Operator4/2
  [VPMM_SysPwrSta_enum] -> Equal3/1
  Equal1/1 -> Logical Operator3/2
  Constant2/1 -> Equal3/2
  Constant1/1 -> Equal1/2
  Equal3/1 -> Logical Operator3/1
  [VPMM_SysPwrSta_enum] -> Equal1/1
  Switch2/1 -> Logical Operator4/1, Logical Operator1/1
  Logical Operator4/1 -> CFS_flg/1
  VPMM_SysPwrSta_enum/1 -> [VPMM_SysPwrSta_enum]
  Constant5/1 -> Equal5/2
  VAPM_SNSRLayout_enum/1 -> Equal5/1
  Equal5/1 -> Switch2/2
  Constant25/1 -> Switch2/3
  USSSta_flg/1 -> Switch2/1

== system ddm/DDM/DDM/APM/Subsystem3 ==
  USSSta_flg : Inport
  VPMM_SysPwrSta_enum : Inport  Port=2
  VAPM_SNSRLayout_enum : Inport  Port=3
  Constant1 : Constant  Value=ENUM_PWRSTASW_READY
  Constant17 : Constant  Value=ENUM_PWRSTASW_READY
  Constant2 : Constant  Value=ENUM_PWRSTASW_ON
  Constant25 : Constant  Value=FALSE
  Constant3 : Constant  Value=ENUM_PWRSTASW_ON
  Constant4 : Constant  Value=ENUM_APS
  Constant5 : Constant  Value=ENUM_PAS_R2F2
  Equal{1..6} (6 alike) : RelationalOperator  Operator===  OutDataTypeStr=boolean  RndMeth=Simplest
  Logical Operator1 : Logic  Operator=NOT  AllPortsSameDT=off  OutDataTypeStr=boolean
  Logical Operator13 : Logic  Operator=OR  AllPortsSameDT=off  OutDataTypeStr=boolean
  Logical Operator2 : Logic  AllPortsSameDT=off  OutDataTypeStr=boolean
  Logical Operator3 : Logic  Operator=OR  AllPortsSameDT=off  OutDataTypeStr=boolean
  Logical Operator4 : Logic  AllPortsSameDT=off  OutDataTypeStr=boolean
  Logical Operator5 : Logic  Operator=OR  AllPortsSameDT=off  OutDataTypeStr=boolean
  Switch2 : Switch  Criteria=u2 ~= 0
  Pass_flg : Outport
  CFS_flg : Outport  Port=2
  wires:
  VPMM_SysPwrSta_enum/1 -> [VPMM_SysPwrSta_enum]
  Logical Operator4/1 -> CFS_flg/1
  Switch2/1 -> Logical Operator4/1, Logical Operator1/1
  [VPMM_SysPwrSta_enum] -> Equal1/1
  Equal3/1 -> Logical Operator3/1
  Constant1/1 -> Equal1/2
  Constant2/1 -> Equal3/2
  Equal1/1 -> Logical Operator3/2
  [VPMM_SysPwrSta_enum] -> Equal3/1
  Logical Operator3/1 -> Logical Operator4/2
  Logical Operator2/1 -> Pass_flg/1
  Logical Operator1/1 -> Logical Operator2/2
  Logical Operator13/1 -> Logical Operator2/1
  [VPMM_SysPwrSta_enum] -> Equal6/1
  Equal2/1 -> Logical Operator13/2
  Constant3/1 -> Equal6/2
  Constant17/1 -> Equal2/2
  Equal6/1 -> Logical Operator13/1
  [VPMM_SysPwrSta_enum] -> Equal2/1
  USSSta_flg/1 -> Switch2/1
  Equal4/1 -> Logical Operator5/1
  Constant25/1 -> Switch2/3
  Constant4/1 -> Equal4/1
  VAPM_SNSRLayout_enum/1 -> Equal4/2, Equal5/1
  Logical Operator5/1 -> Switch2/2
  Equal5/1 -> Logical Operator5/2
  Constant5/1 -> Equal5/2

== system ddm/DDM/DDM/APM/Subsystem4 ==
  USSSta_flg : Inport
  VPMM_SysPwrSta_enum : Inport  Port=2
  VAPM_SNSRLayout_enum : Inport  Port=3
  Constant1 : Constant  Value=ENUM_PWRSTASW_READY
  Constant17 : Constant  Value=ENUM_PWRSTASW_READY
  Constant2 : Constant  Value=ENUM_PWRSTASW_ON
  Constant25 : Constant  Value=FALSE
  Constant3 : Constant  Value=ENUM_PWRSTASW_ON
  Constant5 : Constant  Value=ENUM_APS
  Equal{1..3,5..6} (5 alike) : RelationalOperator  Operator===  OutDataTypeStr=boolean  RndMeth=Simplest
  Logical Operator1 : Logic  Operator=NOT  AllPortsSameDT=off  OutDataTypeStr=boolean
  Logical Operator13 : Logic  Operator=OR  AllPortsSameDT=off  OutDataTypeStr=boolean
  Logical Operator2 : Logic  AllPortsSameDT=off  OutDataTypeStr=boolean
  Logical Operator3 : Logic  Operator=OR  AllPortsSameDT=off  OutDataTypeStr=boolean
  Logical Operator4 : Logic  AllPortsSameDT=off  OutDataTypeStr=boolean
  Switch2 : Switch  Criteria=u2 ~= 0
  Pass_flg : Outport
  CFS_flg : Outport  Port=2
  wires:
  [VPMM_SysPwrSta_enum] -> Equal2/1
  Equal6/1 -> Logical Operator13/1
  Constant17/1 -> Equal2/2
  Constant3/1 -> Equal6/2
  Equal2/1 -> Logical Operator13/2
  [VPMM_SysPwrSta_enum] -> Equal6/1
  Logical Operator13/1 -> Logical Operator2/1
  Logical Operator1/1 -> Logical Operator2/2
  Logical Operator2/1 -> Pass_flg/1
  Logical Operator3/1 -> Logical Operator4/2
  [VPMM_SysPwrSta_enum] -> Equal3/1
  Equal1/1 -> Logical Operator3/2
  Constant2/1 -> Equal3/2
  Constant1/1 -> Equal1/2
  Equal3/1 -> Logical Operator3/1
  [VPMM_SysPwrSta_enum] -> Equal1/1
  Switch2/1 -> Logical Operator4/1, Logical Operator1/1
  Logical Operator4/1 -> CFS_flg/1
  VPMM_SysPwrSta_enum/1 -> [VPMM_SysPwrSta_enum]
  Constant5/1 -> Equal5/2
  VAPM_SNSRLayout_enum/1 -> Equal5/1
  Equal5/1 -> Switch2/2
  Constant25/1 -> Switch2/3
  USSSta_flg/1 -> Switch2/1
